simulink model "APP"  (R2023a)
settings: Solver=FixedStepAuto  StartTime=0.0  StopTime=1  RelTol=1e-3
libraries: simulink x2, pil_lib x1
settings Model: Creator=esabe  LastModifiedBy=esabe
settings OptimizationCC: DefaultParameterBehavior=Inlined  UseDivisionForNetSlopeComputation=on  GainParamInheritBuiltInType=on  UseFloatMulNetSlope=on  InlineInvariantSignals=on  PassReuseOutputArgsAs=Individual arguments  ZeroExternalMemoryAtStartup=off  ZeroInternalMemoryAtStartup=off  NoFixptDivByZeroProtection=on  EfficientFloat2IntCast=on  LifeSpan=1  OptimizeBlockOrder=speed  DifferentSizesBufferReuse=on  EfficientTunableParamExpr=on
settings DebuggingCC: ParameterTunabilityLossMsg=error
settings HardwareCC: ProdBitPerPointer=32  ProdBitPerSizeT=32  ProdBitPerPtrDiffT=32  ProdLargestAtomicInteger=Long  ProdLargestAtomicFloat=Double  ProdWordSize=32  ProdLongLongMode=on  ProdHWDeviceType=ARM Compatible->ARM Cortex-M
settings SFSimCC: MATLABDynamicMemAlloc=off
settings RTWCC: Description=Embedded Coder  SystemTargetFile=ert.tlc  TemplateMakefile=ert_default_tmf
settings CodeAppCC: ForceParamTrailComments=on  IgnoreCustomStorageClasses=off  OperatorAnnotations=on  SimulinkDataObjDesc=on  SFDataObjDesc=on  CustomSymbolStrGlobalVar=rt$N$M  CustomSymbolStrType=$N$M  CustomSymbolStrFcn=$N$M$F  CustomSymbolStrMacro=$N$M  InsertBlockDesc=on
settings ERTTargetCC: TargetLangStandard=C99 (ISO)  GenerateSampleERTMain=on  IncludeMdlTerminateFcn=off  CombineSignalStateStructs=on  SupportComplex=off  SupportContinuousTime=on  SupportNonInlinedSFcns=on  InlinedParameterPlacement=NonHierarchical  ERTCustomFileTemplate=example_file_process.tlc  ERTFilePackagingFormat=CompactWithDataFile

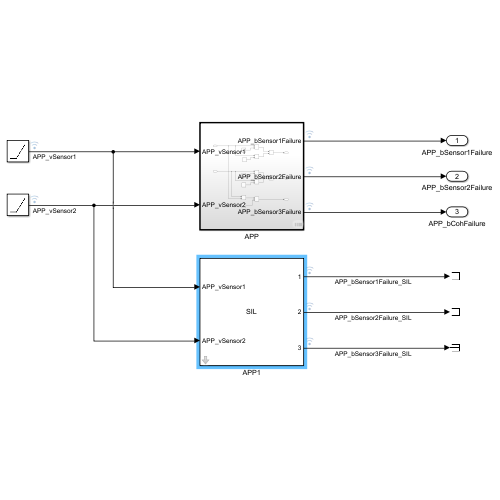
[thumbnail: Simulink's stored preview of the top-level diagram]
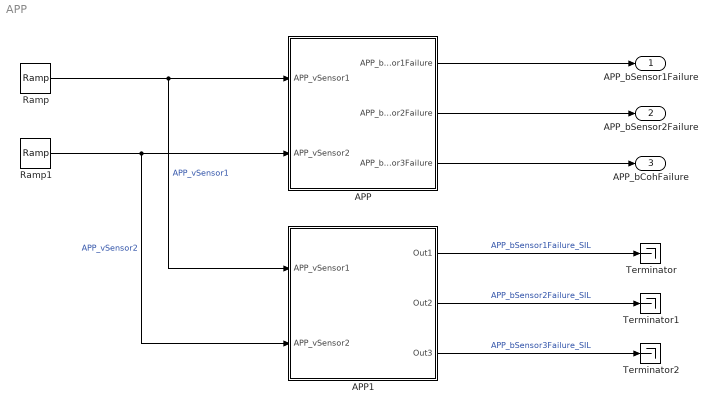
== system APP ==
  APP : Subsystem  TreatAsAtomicUnit=on
      settings: RTWSystemCode=Nonreusable function
  APP1 : Subsystem  Tag=__SL_testing_harness_stub_  DialogController=pil_create_dialog  LoadFcn=|
      | try
      |    if ~strcmp(rtw.pil.getPILVersion, '9.14 (R2023a)_15')
      |       set_param(gcb, 'DialogController', '');
      |       set_param(gcb, 'DialogControllerArgs', '');
      |    end
      | catch e
      |       set_param(gcb, 'DialogController', '');
      |       set_param(gcb, 'DialogControllerArgs', '');
      | end
      mask help: PIL:pil:XILBlockMaskDesc
      mask Display: disp('SIL');
  Ramp : simulink/Sources/Ramp  slope=4  start=0  InitialOutput=0.5
  Ramp1 : simulink/Sources/Ramp  slope=-4  start=0  InitialOutput=4.5
  Terminator : Terminator
  Terminator1 : Terminator
  Terminator2 : Terminator
  APP_bSensor1Failure : Outport
  APP_bSensor2Failure : Outport  Port=2
  APP_bCohFailure : Outport  Port=3
  wires:
  APP/1(APP_bSensor1Failure) -> APP_bSensor1Failure/1
  APP/2(APP_bSensor2Failure) -> APP_bSensor2Failure/1
  APP/3(APP_bSensor3Failure) -> APP_bCohFailure/1
  APP1/3(Out3) -> Terminator2/1  "APP_bSensor3Failure_SIL"
  APP1/2(Out2) -> Terminator1/1  "APP_bSensor2Failure_SIL"
  APP1/1(Out1) -> Terminator/1  "APP_bSensor1Failure_SIL"
  Ramp1/1 -> APP1/2(APP_vSensor2), APP/2(APP_vSensor2)  "APP_vSensor2"
  Ramp/1 -> APP1/1(APP_vSensor1), APP/1(APP_vSensor1)  "APP_vSensor1"

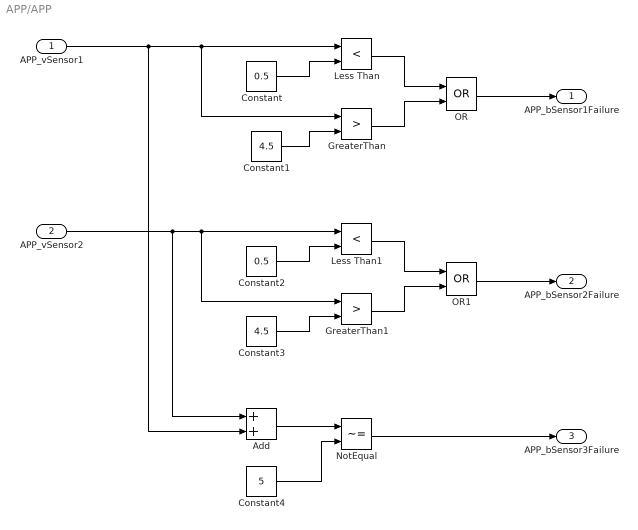
== system APP/APP ==
  APP_vSensor1 : Inport
  APP_vSensor2 : Inport  Port=2
  Add : Sum
  Constant : Constant  Value=0.5
  Constant1 : Constant  Value=4.5
  Constant2 : Constant  Value=0.5
  Constant3 : Constant  Value=4.5
  Constant4 : Constant  Value=5
  GreaterThan : RelationalOperator  Operator=>  OutDataTypeStr=boolean  RndMeth=Simplest  InputSameDT=off
  GreaterThan1 : RelationalOperator  Operator=>  OutDataTypeStr=boolean  RndMeth=Simplest  InputSameDT=off
  Less Than : RelationalOperator  Operator=<  OutDataTypeStr=boolean  RndMeth=Simplest  InputSameDT=off
  Less Than1 : RelationalOperator  Operator=<  OutDataTypeStr=boolean  RndMeth=Simplest  InputSameDT=off
  NotEqual : RelationalOperator  Operator=~=  OutDataTypeStr=boolean  RndMeth=Simplest  InputSameDT=off
  OR : Logic  Operator=OR  AllPortsSameDT=off  OutDataTypeStr=boolean
  OR1 : Logic  Operator=OR  AllPortsSameDT=off  OutDataTypeStr=boolean
  APP_bSensor1Failure : Outport
  APP_bSensor2Failure : Outport  Port=2
  APP_bSensor3Failure : Outport  Port=3
  wires:
  APP_vSensor1/1 -> Add/2, GreaterThan/1, Less Than/1
  Constant1/1 -> GreaterThan/2
  GreaterThan1/1 -> OR1/2
  Less Than/1 -> OR/1
  Constant/1 -> Less Than/2
  GreaterThan/1 -> OR/2
  APP_vSensor2/1 -> Add/1, GreaterThan1/1, Less Than1/1
  Constant3/1 -> GreaterThan1/2
  Constant2/1 -> Less Than1/2
  Less Than1/1 -> OR1/1
  Add/1 -> NotEqual/1
  Constant4/1 -> NotEqual/2
  OR/1 -> APP_bSensor1Failure/1
  OR1/1 -> APP_bSensor2Failure/1
  NotEqual/1 -> APP_bSensor3Failure/1

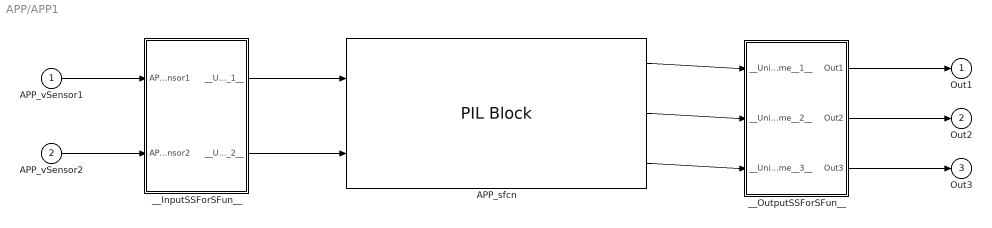
== system APP/APP1 ==
  APP_vSensor1 : Inport
  APP_vSensor2 : Inport  Port=2
  APP_sfcn : pil_lib/PIL Block  SimulationMode=SIL  IsTopModelPIL=off  CodeDir=APP0_ert_rtw  AnchorDir=C:\Users\esabe\Downloads  ConfigName=Software-in-the-Loop (SIL)  XrelIsTopModelCode=on  XrelIsReusable=off  XrelDWorkNames={}  XrelDWorkTypes={}  XrelModelArgVals={}  XrelOrderedParamNames={}
  __InputSSForSFun__ : Subsystem
  __OutputSSForSFun__ : Subsystem
  Out1 : Outport
  Out2 : Outport  Port=2
  Out3 : Outport  Port=3
  wires:
  __OutputSSForSFun__/3(Out3) -> Out3/1
  __OutputSSForSFun__/2(Out2) -> Out2/1
  __OutputSSForSFun__/1(Out1) -> Out1/1
  APP_sfcn/3 -> __OutputSSForSFun__/3(__UniqueInportName__3__)
  APP_sfcn/2 -> __OutputSSForSFun__/2(__UniqueInportName__2__)
  APP_sfcn/1 -> __OutputSSForSFun__/1(__UniqueInportName__1__)
  __InputSSForSFun__/2(__UniqueOutportName__2__) -> APP_sfcn/2
  __InputSSForSFun__/1(__UniqueOutportName__1__) -> APP_sfcn/1
  APP_vSensor2/1 -> __InputSSForSFun__/2(APP_vSensor2)
  APP_vSensor1/1 -> __InputSSForSFun__/1(APP_vSensor1)

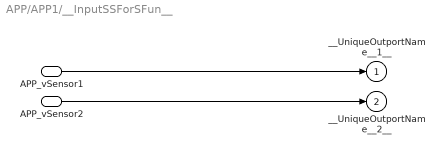
== system APP/APP1/__InputSSForSFun__ ==
  APP_vSensor1 : Inport
  APP_vSensor2 : Inport  Port=2
  __UniqueOutportName__1__ : Outport
  __UniqueOutportName__2__ : Outport  Port=2
  wires:
  APP_vSensor2/1 -> __UniqueOutportName__2__/1
  APP_vSensor1/1 -> __UniqueOutportName__1__/1

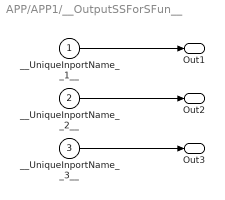
== system APP/APP1/__OutputSSForSFun__ ==
  __UniqueInportName__1__ : Inport
  __UniqueInportName__2__ : Inport  Port=2
  __UniqueInportName__3__ : Inport  Port=3
  Out1 : Outport
  Out2 : Outport  Port=2
  Out3 : Outport  Port=3
  wires:
  __UniqueInportName__3__/1 -> Out3/1
  __UniqueInportName__2__/1 -> Out2/1
  __UniqueInportName__1__/1 -> Out1/1
